simulink model "verify_Thermosyphon_mdl"  (R2016b)
settings: Solver=ode45  StartTime=0.0  StopTime=200  MaxStep=5  RelTol=1e-3  EnableMultiTasking=on
libraries: carnot x5
settings Model: Creator=drhf  LastModifiedBy=drhf
settings DataIOCC: SaveFormat=Array  SignalLoggingSaveFormat=ModelDataLogs
settings OptimizationCC: ExpressionDepthLimit=2147483647  LifeSpan=inf
settings DebuggingCC: UnderspecifiedInitializationDetection=Classic  MergeDetectMultiDrivingBlocksExec=none  SolverPrmCheckMsg=warning  FcnCallInpInsideContextMsg=warning  StateNameClashWarn=warning  SFUnexpectedBacktrackingDiag=warning  SFNoUnconditionalDefaultTransitionDiag=warning  SFExecutionAtInitializationDiag=none
settings HardwareCC: ProdBitPerPointer=32  ProdBitPerSizeT=32  ProdBitPerPtrDiffT=32  ProdLargestAtomicFloat=None  ProdIntDivRoundTo=Undefined  ProdEndianess=Unspecified  ProdWordSize=32  ProdHWDeviceType=32-bit Generic
settings ModelReferenceCC: PropagateSignalLabelsOutOfModel=off
settings GRTTargetCC: TargetLangStandard=C89/C90 (ANSI)  GeneratePreprocessorConditionals=Disable all  CombineOutputUpdateFcns=off  GRTInterface=on
settings ConfigComp: CovMetricSettings=dw  CovHtmlReporting=on  CovSaveCumulativeToWorkspaceVar=on  CovSaveSingleToWorkspaceVar=on  CovExternalEMLEnable=off

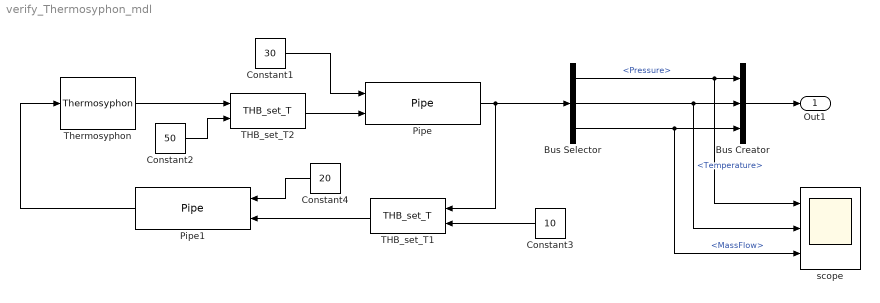
== system verify_Thermosyphon_mdl ==
  Bus Creator : BusCreator  Inputs=3
  Bus Selector : BusSelector  OutputSignals=Pressure,Temperature,MassFlow
  Constant1 : Constant  Value=30
  Constant2 : Constant  Value=50
  Constant3 : Constant  Value=10
  Constant4 : Constant  Value=20
  Pipe : carnot/Hydraulics/Pipe  dia=0.02  len=10  hgt=5  uloss=100/20/10  cond=0  cwall=1000  t0=20  lin=100/0.2  qua=100/0.2^2  nodes=10
  Pipe1 : carnot/Hydraulics/Pipe  dia=0.02  len=10  hgt=-5  uloss=100/20/10  cond=0  cwall=1000  t0=20  lin=100/0.2  qua=100/0.2^2  nodes=10
  THB_set_T1 : carnot/Source/Simple/THB_set_T
  THB_set_T2 : carnot/Source/Simple/THB_set_T
  Thermosyphon : carnot/Hydraulics/Thermosyphon  dia=0.025  fluid_id=Water  mix=0  mix2=0  mix3=0  p0=2e5  t1=5
  scope : Scope  NumInputPorts=3
  Out1 : Outport
  wires:
  Bus Creator/1 -> Out1/1
  Bus Selector/3 -> scope/3, Bus Creator/3  "<MassFlow>"
  Bus Selector/1 -> scope/1, Bus Creator/1  "<Pressure>"
  Bus Selector/2 -> scope/2, Bus Creator/2  "<Temperature>"
  Pipe1/1 -> Thermosyphon/1
  Thermosyphon/1 -> THB_set_T2/1
  THB_set_T2/1 -> Pipe/2
  Constant1/1 -> Pipe/1
  Constant2/1 -> THB_set_T2/2
  THB_set_T1/1 -> Pipe1/2
  Pipe/1 -> Bus Selector/1, THB_set_T1/1
  Constant3/1 -> THB_set_T1/2
  Constant4/1 -> Pipe1/1
